simulink model "nanogrid_model"  (R2022a)
settings: Solver=VariableStepAuto  StartTime=0.0  StopTime=86000  RelTol=1e-3
undefined symbols (not defined in the file): Ion, Lithium, sigbuilder_block
libraries: spsCurrentMeasurementLib x18, spsControlledCurrentSourceLib x16, spsVoltageMeasurementLib x12, spsParallelRLCBranchLib x2, spsVariableResistorLib x2, spsBatteryLib x2, spsPVArrayLib x2, spsControlledVoltageSourceLib x1, spsSeriesRLCBranchLib x1, spspowerguiLib x1
(part 2 of 2)

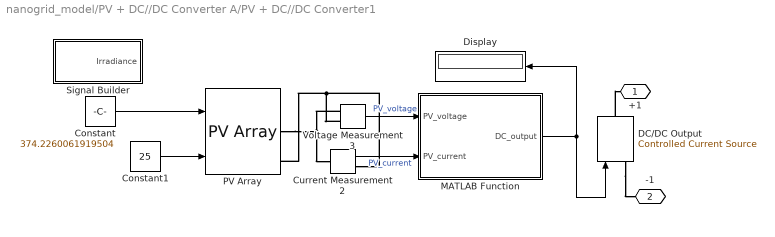
== system nanogrid_model/PV + DC//DC Converter A/PV + DC//DC Converter1 ==
  Constant : Constant  Value=374.2260061919504
  Constant1 : Constant  Value=25
  Current Measurement2 : spsCurrentMeasurementLib/Current Measurement  PhasorSimulation=off  OutputType=Complex  PSBequivalent=0
  DC/DC Output : spsControlledCurrentSourceLib/Controlled Current Source  Initialize=on  Source_Type=DC  Amplitude=0  Phase=0  Frequency=0  Measurements=None
  Display : Display
  MATLAB Function : MATLAB Function  TreatAsAtomicUnit=on
  PV Array : spsPVArrayLib/PV Array  Npar=40  Nser=10  PlotType=array @ 1000 W/m2 & specified temperatures  S_vec="[ 1000  500  100 ]"  Temp_C_vec="[ 45 25  ]"  ModuleName=User-defined  PlotWhenSelected=off  Pm=213.15  Ncell=60  Voc=36.3  Isc=7.84  Vm=29  Im=7.35  beta_Voc_pc=-0.36099  alpha_Isc_pc=0.102  beta_Voc=-0.13104  alpha_Isc=0.0079968  IL=7.8654  I0=2.9273e-10  nI=0.98119  Rsh=313.0553  Rs=0.39381  RobustModel=off  RobustCellTemperature=313.3991  BAL=on  Tc=1e-6  Tfilter=5e-5
  Signal Builder : Subsystem  Tag=STV Subsys  LoadFcn=sigbuilder_block('load');  StartFcn=sigbuilder_block('start');  StopFcn=sigbuilder_block('stop');  ClipboardFcn=sigbuilder_block('clipboard');  mask(Sigbuilder block){tuvar=[0:10]}
      mask help: Simulink:masks:SigbuilderBlock_MD
      mask init:
      | if ~strcmp(get_param(bdroot(gcbh),'SimulationStatus'),'stopped') tuvar = sigbuilder_block('maskInit'); end
      settings: CopyFcn=sigbuilder_block('copy');  DeleteFcn=sigbuilder_block('delete');  ModelCloseFcn=sigbuilder_block('modelClose');  PreSaveFcn=sigbuilder_block('preSave');  PauseFcn=sigbuilder_block('pause');  ContinueFcn=sigbuilder_block('continue');  NameChangeFcn=sigbuilder_block('namechange');  OpenFcn=sigbuilder_block('open',[509.4 101.4 550.8 400.2 ]);  CloseFcn=sigbuilder_block('close');
      mask Display: plot(0, 0, 100, 100,[2, 2, 32, 32, 2], [68, 8, 8, 68, 68],[32, 2], [38, 38], [32, 19, 2],[53, 60, 44], [32, 17, 17, 2],[16, 16, 31, 31]);txt = getActiveGroup(gcbh);text(2, 100, txt,'verticalAlignment', 'top');
  Voltage Measurement3 : spsVoltageMeasurementLib/Voltage Measurement  PhasorSimulation=off  OutputType=Complex  PSBequivalent=0
  +1 : PMIOPort  Side=Right
  -1 : PMIOPort  Port=2  Side=Right
  wires:
  MATLAB Function/1(DC_output) -> DC/DC Output/1, Display/1
  Voltage Measurement3/1 -> MATLAB Function/1(PV_voltage)  "PV_voltage"
  Current Measurement2/1 -> MATLAB Function/2(PV_current)  "PV_current"
  Constant1/1 -> PV Array/2
  Constant/1 -> PV Array/1
  connections:
  DC/DC Output/LConn1 -- -1/RConn1
  PV Array/RConn1 -- Voltage Measurement3/LConn1 -- Current Measurement2/LConn1
  Current Measurement2/RConn1 -- PV Array/RConn2 -- Voltage Measurement3/LConn2
  DC/DC Output/RConn1 -- +1/RConn1

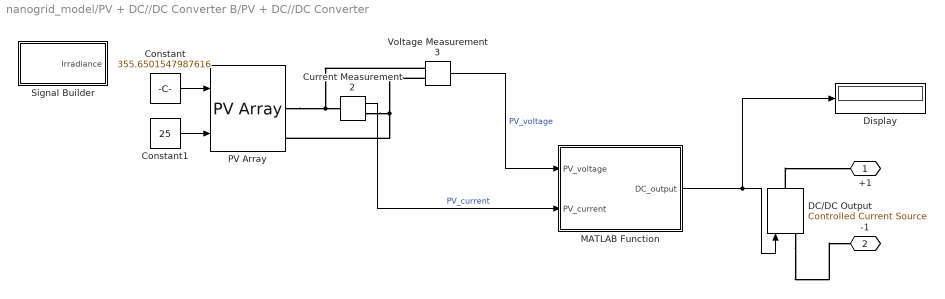
== system nanogrid_model/PV + DC//DC Converter B/PV + DC//DC Converter ==
  Constant : Constant  Value=355.6501547987616
  Constant1 : Constant  Value=25
  Current Measurement2 : spsCurrentMeasurementLib/Current Measurement  PhasorSimulation=off  OutputType=Complex  PSBequivalent=0
  DC/DC Output : spsControlledCurrentSourceLib/Controlled Current Source  Initialize=on  Source_Type=DC  Amplitude=0  Phase=0  Frequency=0  Measurements=None
  Display : Display
  MATLAB Function : MATLAB Function  TreatAsAtomicUnit=on
  PV Array : spsPVArrayLib/PV Array  Npar=40  Nser=10  PlotType=array @ 1000 W/m2 & specified temperatures  S_vec="[ 1000  500  100 ]"  Temp_C_vec="[ 45 25  ]"  ModuleName=User-defined  PlotWhenSelected=off  Pm=213.15  Ncell=60  Voc=36.3  Isc=7.84  Vm=29  Im=7.35  beta_Voc_pc=-0.36099  alpha_Isc_pc=0.102  beta_Voc=-0.13104  alpha_Isc=0.0079968  IL=7.8654  I0=2.9273e-10  nI=0.98119  Rsh=313.0553  Rs=0.39381  RobustModel=off  RobustCellTemperature=313.3991  BAL=on  Tc=1e-6  Tfilter=5e-5
  Signal Builder : Subsystem  Tag=STV Subsys  LoadFcn=sigbuilder_block('load');  StartFcn=sigbuilder_block('start');  StopFcn=sigbuilder_block('stop');  ClipboardFcn=sigbuilder_block('clipboard');  mask(Sigbuilder block){tuvar=[0:10]}
      mask help: Simulink:masks:SigbuilderBlock_MD
      mask init:
      | if ~strcmp(get_param(bdroot(gcbh),'SimulationStatus'),'stopped') tuvar = sigbuilder_block('maskInit'); end
      settings: CopyFcn=sigbuilder_block('copy');  DeleteFcn=sigbuilder_block('delete');  ModelCloseFcn=sigbuilder_block('modelClose');  PreSaveFcn=sigbuilder_block('preSave');  PauseFcn=sigbuilder_block('pause');  ContinueFcn=sigbuilder_block('continue');  NameChangeFcn=sigbuilder_block('namechange');  OpenFcn=sigbuilder_block('open',[509.4 101.4 550.8 400.2 ]);  CloseFcn=sigbuilder_block('close');
      mask Display: plot(0, 0, 100, 100,[2, 2, 32, 32, 2], [68, 8, 8, 68, 68],[32, 2], [38, 38], [32, 19, 2],[53, 60, 44], [32, 17, 17, 2],[16, 16, 31, 31]);txt = getActiveGroup(gcbh);text(2, 100, txt,'verticalAlignment', 'top');
  Voltage Measurement3 : spsVoltageMeasurementLib/Voltage Measurement  PhasorSimulation=off  OutputType=Complex  PSBequivalent=0
  +1 : PMIOPort  Side=Right
  -1 : PMIOPort  Port=2  Side=Right
  wires:
  MATLAB Function/1(DC_output) -> Display/1, DC/DC Output/1
  Voltage Measurement3/1 -> MATLAB Function/1(PV_voltage)  "PV_voltage"
  Current Measurement2/1 -> MATLAB Function/2(PV_current)  "PV_current"
  Constant1/1 -> PV Array/2
  Constant/1 -> PV Array/1
  connections:
  DC/DC Output/LConn1 -- -1/RConn1
  PV Array/RConn1 -- Voltage Measurement3/LConn1 -- Current Measurement2/LConn1
  Current Measurement2/RConn1 -- PV Array/RConn2 -- Voltage Measurement3/LConn2
  DC/DC Output/RConn1 -- +1/RConn1

== system nanogrid_model/AC+DC Load & DC//AC Converter A/AC+DC Load & DC//AC Converter1/Signal Builder ==
  Demux : Demux  Tag=STV Demux  Outputs=1
      settings: DisplayOption=none
  FromWs : FromWorkspace  Tag=STV FromWs  VariableName=tuvar
      SigBuilderData=|
      | common.afterFinalStr = 'Extrapolate'
      | common.sampleTime = 0
      | dataSet.timeRange = [0 82411]
      | dataSet.name = 'Sheet1'
      | sbobj.Groups.Name = 'Sheet1'
      | sbobj.Groups.Signals.Name = 'Load'
      | sbobj.Groups.Signals.XData = [0 3583 7166 10750 14332 17915 21498 25083 28666 32249 35832 39415 42998 46581 50164 53747 57330 60913 65000 68079 71662 75245 78828 82411]
      | sbobj.Groups.Signals.YData = [10 10 10 10 10 10 50 70 90 20 20 20 20 20 20 20 20 50 70 90 100 100 100 50]
  Load : Outport  Tag=STV Outport
  wires:
  Demux/1 -> Load/1
  FromWs/1 -> Demux/1

== system nanogrid_model/AC//DC Load & DC//AC Converter B/AC//DC Load & DC//AC Converter/Signal Builder ==
  Demux : Demux  Tag=STV Demux  Outputs=1
      settings: DisplayOption=none
  FromWs : FromWorkspace  Tag=STV FromWs  VariableName=tuvar
      SigBuilderData=|
      | common.afterFinalStr = 'Extrapolate'
      | common.sampleTime = 0
      | dataSet.timeRange = [0 82411]
      | dataSet.name = 'Sheet1'
      | sbobj.Groups.Name = 'Sheet1'
      | sbobj.Groups.Signals.Name = 'Load'
      | sbobj.Groups.Signals.XData = [0 3583 7166 10750 14332 17915 21498 25083 28666 32249 35832 39415 42998 46581 50164 53747 57330 60913 65000 68079 71662 75245 78828 82411]
      | sbobj.Groups.Signals.YData = [62 81 91 84.5 81 76 61 70 90 76.5 58 71.5 54.5 68.5 60.5 73.5 64.5 69.5 70 90 100 100 100 50]
      | sbobj.Groups.TimeRange = [0 82411]
  Load : Outport  Tag=STV Outport
  wires:
  Demux/1 -> Load/1
  FromWs/1 -> Demux/1

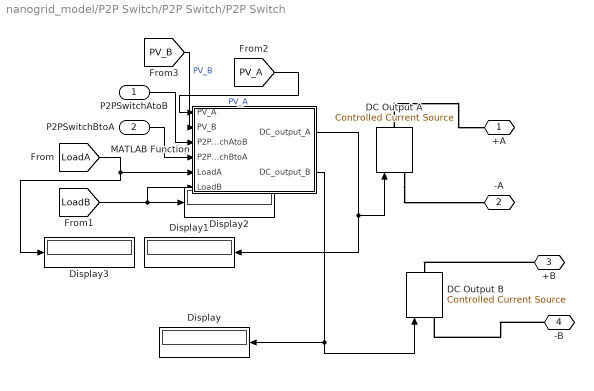
== system nanogrid_model/P2P Switch/P2P Switch/P2P Switch ==
  P2PSwitchAtoB : Inport
  P2PSwitchBtoA : Inport  Port=2
  DC Output A : spsControlledCurrentSourceLib/Controlled Current Source  Initialize=on  Source_Type=DC  Amplitude=0  Phase=0  Frequency=0  Measurements=None
  DC Output B : spsControlledCurrentSourceLib/Controlled Current Source  Initialize=on  Source_Type=DC  Amplitude=0  Phase=0  Frequency=0  Measurements=None
  Display{,1..3} (4 alike) : Display
  MATLAB Function : MATLAB Function  TreatAsAtomicUnit=on
  +A : PMIOPort  Side=Right
  -A : PMIOPort  Port=2  Side=Right
  +B : PMIOPort  Port=3  Side=Right
  -B : PMIOPort  Port=4  Side=Right
  wires:
  MATLAB Function/1(DC_output_A) -> DC Output A/1, Display1/1
  P2PSwitchAtoB/1 -> MATLAB Function/3(P2PSwitchAtoB)
  MATLAB Function/2(DC_output_B) -> Display/1, DC Output B/1
  P2PSwitchBtoA/1 -> MATLAB Function/4(P2PSwitchBtoA)
  [LoadA] -> Display3/1, MATLAB Function/5(LoadA)
  [LoadB] -> Display2/1, MATLAB Function/6(LoadB)
  [PV_A] -> MATLAB Function/1(PV_A)  "PV_A"
  [PV_B] -> MATLAB Function/2(PV_B)  "PV_B"
  connections:
  DC Output A/LConn1 -- -A/RConn1
  DC Output A/RConn1 -- +A/RConn1
  +B/RConn1 -- DC Output B/RConn1
  -B/RConn1 -- DC Output B/LConn1

== system nanogrid_model/PV + DC//DC Converter A/PV + DC//DC Converter1/Signal Builder ==
  Demux : Demux  Tag=STV Demux  Outputs=1
      settings: DisplayOption=none
  FromWs : FromWorkspace  Tag=STV FromWs  VariableName=tuvar
      SigBuilderData=|
      | common.afterFinalStr = 'Extrapolate'
      | common.sampleTime = 0
      | dataSet.timeRange = [0 82411]
      | dataSet.name = 'Sheet1'
      | sbobj.Groups.Name = 'Sheet1'
      | sbobj.Groups.Signals.Name = 'Irradiance'
      | sbobj.Groups.Signals.XData = [0 3583 7166 10750 14332 17915 21498 25083 28666 32249 35832 39415 42998 46581 50164 53747 57330 60913 65000 68079 71662 75245 78828 82411]
      | sbobj.Groups.Signals.YData = [0 0 0 0 0 0 0 100 200 300 400 500 600 500 400 300 200 100 0 0 0 0 0 0]
      | sbobj.Groups.TimeRange = [0 86000]
  Irradiance : Outport  Tag=STV Outport
  wires:
  Demux/1 -> Irradiance/1
  FromWs/1 -> Demux/1

== system nanogrid_model/PV + DC//DC Converter B/PV + DC//DC Converter/Signal Builder ==
  Demux : Demux  Tag=STV Demux  Outputs=1
      settings: DisplayOption=none
  FromWs : FromWorkspace  Tag=STV FromWs  VariableName=tuvar
      SigBuilderData=|
      | common.afterFinalStr = 'Extrapolate'
      | common.sampleTime = 0
      | dataSet.timeRange = [0 82411]
      | dataSet.name = 'Sheet1'
      | sbobj.Groups.Name = 'Sheet1'
      | sbobj.Groups.Signals.Name = 'Irradiance'
      | sbobj.Groups.Signals.XData = [0 3583 7166 10750 14332 17915 21498 25083 28666 32249 35832 39415 42998 46581 50164 53747 57330 60913 65000 68079 71662 75245 78828 82411]
      | sbobj.Groups.Signals.YData = [0 0 0 0 0 0 0 100 200 300 400 500 600 500 400 300 200 100 0 0 0 0 0 0]
      | sbobj.Groups.TimeRange = [0 86000]
  Irradiance : Outport  Tag=STV Outport
  wires:
  Demux/1 -> Irradiance/1
  FromWs/1 -> Demux/1

== stateflow chart nanogrid_model/Stateflow Algorithm A ==
  state PurchaseEnergy
    exit:
    switchUtilityPurchase=0;
    P2PPurchaseRequest=0;
    state Utilitygrid
      entry:
      currentState = "PUG";
    state NanoGrid
      entry:
      currentState = "PNG";
    PurchaseEnergy.Utilitygrid -> (junction 309) : [DERPrice<=gridPrice || gridOutage]
    (junction 309) -> PurchaseEnergy.Utilitygrid [order 2] : {P2PPurchaseRequest=0;switchUtilityPurchase=1;}
    (junction 310) -> PurchaseEnergy.Utilitygrid [order 1] : [~P2PEnergyTrading]{switchUtilityPurchase=1;}
    (default) -> (junction 307)
    (junction 307) -> (junction 309)
    (junction 310) -> (junction 309) [order 3]
    (junction 308) -> (junction 310) : {P2PPurchaseRequest=1;}
    (junction 309) -> (junction 308) [order 1] : [DERPrice <= gridPrice || gridOutage]
    PurchaseEnergy.NanoGrid -> (junction 309) : [~P2PEnergyTrading||DERPrice>gridPrice]
    (junction 310) -> PurchaseEnergy.NanoGrid [order 2] : [P2PEnergyTrading]{switchUtilityPurchase=0;}
  state SellEnergy
    exit:
    switchUtilitySell=0;
    P2PSaleRequest=0;
    state Utilitygrid
      entry:
      currentState = "SUG";
    state NanoGrid
      entry:
      currentState = "SNG";
    (junction 325) -> SellEnergy.Utilitygrid [order 2] : {P2PSaleRequest=0;switchUtilitySell=1;}
    SellEnergy.Utilitygrid -> (junction 325) : [gridOutage||DERPrice>=feedInTariff]
    (junction 324) -> SellEnergy.Utilitygrid [order 2] : [~P2PEnergyTrading]{switchUtilitySell=1;}
    (default) -> (junction 317)
    (junction 317) -> (junction 325)
    (junction 324) -> (junction 325) [order 3]
    (junction 325) -> (junction 316) [order 1] : [DERPrice >= feedInTariff || gridOutage]
    (junction 316) -> (junction 324) : {P2PSaleRequest=1;}
    SellEnergy.NanoGrid -> (junction 325) : [~P2PEnergyTrading||DERPrice<feedInTariff]
    (junction 324) -> SellEnergy.NanoGrid [order 1] : [P2PEnergyTrading]{switchUtilitySell=0;}
  state SelfConsumption
    state GeneratorMode
      entry:
      currentState = "GM"
      switchGenerator = 1;
      exit:
      switchGenerator = 0;
    state RenewableSources
      entry:
      currentState = "PV"
    (default) -> (junction 281)
    (junction 281) -> GeneratorMode [order 1] : [SOC<=1]
    (junction 281) -> RenewableSources [order 2]
  (default) -> (junction 290)
  (junction 290) -> PurchaseEnergy [order 1] : [SOC<20 && SOC>1]
  (junction 290) -> SellEnergy [order 2] : [SOC>80]
  PurchaseEnergy -> (junction 290) : [SOC>=20 || SOC < 1]
  SellEnergy -> (junction 290) : [SOC<=80]
  SelfConsumption -> (junction 290) : [SOC>80 || SOC<80 && SOC > 1]
  (junction 290) -> SelfConsumption [order 3]
  data: gridOutage input; SOC input; currentState output; DERPrice input; feedInTariff input; switchGenerator output; gridPrice input; switchUtilityPurchase output; switchUtilitySell output; P2PEnergyTrading input; P2PPurchaseRequest output; P2PSaleRequest output

== matlab function nanogrid_model/AC//DC Converter B/MATLAB Function ==
  data: switchGridPurchase input; switchGridSell input; gridOutage input; DC_output output; AC_output output; LoadB input; PV_B input
function [DC_output,AC_output] = fcn(switchGridPurchase, switchGridSell, gridOutage, LoadB, PV_B)

dischargeCurrent = 217;
chargeCurrent = 217;
lowChargeCRate = 0.1;
converterEfficiencyLoss = 0.95;

if(gridOutage)
    DC_output = 0;
    AC_output = 0;
elseif(switchGridSell)
    DC_output = -(dischargeCurrent+PV_B)*converterEfficiencyLoss;
    AC_output = (dischargeCurrent+PV_B)*sqrt(2)*converterEfficiencyLoss;
elseif(switchGridPurchase)
    DC_output = (chargeCurrent*lowChargeCRate+(-LoadB)-PV_B)*converterEfficiencyLoss*1.1;
    AC_output = (-chargeCurrent*lowChargeCRate+(-LoadB)-PV_B)*converterEfficiencyLoss*1.1;
else
    DC_output = 0;
    AC_output = 0; 
end
end

== stateflow chart nanogrid_model/Stateflow Algorithm B ==
  state PurchaseEnergy
    exit:
    switchUtilityPurchase=0;
    P2PPurchaseRequest=0;
    state Utilitygrid
      entry:
      currentState = "PUG";
    state NanoGrid
      entry:
      currentState = "PNG";
    PurchaseEnergy.Utilitygrid -> (junction 705) : [DERPrice<=gridPrice || gridOutage]
    (junction 705) -> PurchaseEnergy.Utilitygrid [order 2] : {P2PPurchaseRequest=0;switchUtilityPurchase=1;}
    (junction 702) -> PurchaseEnergy.Utilitygrid [order 1] : [~P2PEnergyTrading]{switchUtilityPurchase=1;}
    (default) -> (junction 704)
    (junction 704) -> (junction 705)
    (junction 702) -> (junction 705) [order 3]
    (junction 700) -> (junction 702) : {P2PPurchaseRequest=1;}
    (junction 705) -> (junction 700) [order 1] : [DERPrice <= gridPrice || gridOutage]
    PurchaseEnergy.NanoGrid -> (junction 705) : [~P2PEnergyTrading||DERPrice>gridPrice]
    (junction 702) -> PurchaseEnergy.NanoGrid [order 2] : [P2PEnergyTrading]{switchUtilityPurchase=0;}
  state SellEnergy
    exit:
    switchUtilitySell=0;
    P2PSaleRequest=0;
    state Utilitygrid
      entry:
      currentState = "SUG";
    state NanoGrid
      entry:
      currentState = "SNG";
    (junction 726) -> SellEnergy.Utilitygrid [order 2] : {P2PSaleRequest=0;switchUtilitySell=1;}
    SellEnergy.Utilitygrid -> (junction 726) : [gridOutage||DERPrice>=feedInTariff]
    (junction 742) -> SellEnergy.Utilitygrid [order 2] : [~P2PEnergyTrading]{switchUtilitySell=1;}
    (default) -> (junction 740)
    (junction 740) -> (junction 726)
    (junction 742) -> (junction 726) [order 3]
    (junction 726) -> (junction 738) [order 1] : [DERPrice >= feedInTariff || gridOutage]
    (junction 738) -> (junction 742) : {P2PSaleRequest=1;}
    SellEnergy.NanoGrid -> (junction 726) : [~P2PEnergyTrading||DERPrice<feedInTariff]
    (junction 742) -> SellEnergy.NanoGrid [order 1] : [P2PEnergyTrading]{switchUtilitySell=0;}
  state SelfConsumption
    state GeneratorMode
      entry:
      currentState = "GM"
      switchGenerator = 1;
      exit:
      switchGenerator = 0;
    state RenewableSources
      entry:
      currentState = "PV"
    (default) -> (junction 724)
    (junction 724) -> GeneratorMode [order 1] : [SOC<=1]
    (junction 724) -> RenewableSources [order 2]
  (default) -> (junction 744)
  (junction 744) -> PurchaseEnergy [order 1] : [SOC<20 && SOC>1]
  (junction 744) -> SellEnergy [order 2] : [SOC>80]
  PurchaseEnergy -> (junction 744) : [SOC>=20 || SOC < 1]
  SellEnergy -> (junction 744) : [SOC<=80]
  SelfConsumption -> (junction 744) : [SOC>80 || SOC<80 && SOC > 1]
  (junction 744) -> SelfConsumption [order 3]
  data: gridOutage input; SOC input; currentState output; DERPrice input; feedInTariff input; switchGenerator output; gridPrice input; P2PPurchaseRequest output; P2PSaleRequest output; switchUtilityPurchase output; switchUtilitySell output; P2PEnergyTrading input

== matlab function nanogrid_model/PV + DC//DC Converter B/PV + DC//DC Converter/MATLAB Function ==
  data: PV_voltage input; PV_current input; DC_output output
function DC_output = fcn(PV_voltage, PV_current)

converterEfficiencyLoss = 0.95;

DC_output = PV_current*converterEfficiencyLoss;


end

== matlab function nanogrid_model/Backup Gas Generator + DC//DC Converter B/Backup Gas Generator + DC//DC Converter/MATLAB Function ==
  data: switchGenerator input; Gen_voltage input; Gen_current input; DC_output output; DC_output_Gen output
function [DC_output,DC_output_Gen] = fcn(switchGenerator, Gen_voltage, Gen_current)

converterEfficiencyLoss = 0.95;

if(switchGenerator)
    DC_output_Gen = 200*converterEfficiencyLoss;
else
    DC_output_Gen = 0;
end
DC_output = DC_output_Gen*converterEfficiencyLoss;

== matlab function nanogrid_model/AC//DC Load & DC//AC Converter B/AC//DC Load & DC//AC Converter/MATLAB Function ==
  data: DC_voltage input; DC_current input; AC_output output
function AC_output = fcn(DC_voltage, DC_current)

converterEfficiencyLoss = 0.95;
DC_power = DC_current * DC_voltage;

AC_output = sqrt(2)*converterEfficiencyLoss*DC_current; 

end

== matlab function nanogrid_model/P2P Switch/P2P Switch/P2P Switch/MATLAB Function ==
  data: PV_A input; PV_B input; P2PSwitchAtoB input; DC_output_A output; DC_output_B output; P2PSwitchBtoA input; LoadA input; LoadB input
function [DC_output_A, DC_output_B] = fcn(PV_A, PV_B, P2PSwitchAtoB,P2PSwitchBtoA, LoadA, LoadB)

chargeCurrent = 217;
lowChargeCRate = 0.1;%low c-rates extend battery life cycles
converterEfficiencyLoss = 0.95;

if(P2PSwitchAtoB)
    DC_output_A = -(chargeCurrent*lowChargeCRate*1.1+(-LoadB)-PV_B)*converterEfficiencyLoss;%subtraction of nano grid member b's PV is due to the battery's charge limitation (whatever is produced by the PV does not need to be drawn from A's battery, if the total power would exceed the maximum battery charge current)
    DC_output_B = (chargeCurrent*lowChargeCRate*1.1+(-LoadB)-PV_B)*converterEfficiencyLoss;
elseif(P2PSwitchBtoA)
    DC_output_A = (chargeCurrent*lowChargeCRate*1.1+(-LoadA)-PV_A)*converterEfficiencyLoss;%current must be at least sufficient to supply the load otherwise the battery won't charge
    DC_output_B = -(chargeCurrent*lowChargeCRate*1.1+(-LoadA)-PV_A)*converterEfficiencyLoss;
else
    DC_output_A = 0;
    DC_output_B = 0;
end

== matlab function nanogrid_model/AC//DC Converter A/MATLAB Function ==
  data: switchGridPurchase input; switchGridSell input; DC_output output; AC_output output; gridOutage input; LoadA input; PV_A input
function [DC_output,AC_output] = fcn(switchGridPurchase, switchGridSell, gridOutage, LoadA, PV_A)

dischargeCurrent = 217;
chargeCurrent = 217;
lowChargeCRate = 0.1;
converterEfficiencyLoss = 0.95;

if(gridOutage)
    DC_output = 0;
    AC_output = 0;
elseif(switchGridSell)
    DC_output = -(dischargeCurrent+PV_A);
    AC_output = (dischargeCurrent+PV_A)*sqrt(2);
elseif(switchGridPurchase)
    DC_output = (chargeCurrent*lowChargeCRate*1.1+(-LoadA)-PV_A)*converterEfficiencyLoss;
    AC_output = (-chargeCurrent*lowChargeCRate*1.1+(-LoadA)-PV_A)*converterEfficiencyLoss;
else
    DC_output = 0;
    AC_output = 0; 
end
end

== matlab function nanogrid_model/Backup Gas Generator + DC//DC Converter A/Backup Gas Generator + DC//DC Converter1/MATLAB Function ==
  data: switchGenerator input; DC_output output; DC_output_Gen output
function [DC_output,DC_output_Gen] = fcn(switchGenerator)

converterEfficiencyLoss = 0.95;

if(switchGenerator)
    DC_output_Gen = 200*converterEfficiencyLoss;
else
    DC_output_Gen = 0;
end
DC_output = DC_output_Gen*converterEfficiencyLoss;

== matlab function nanogrid_model/PV + DC//DC Converter A/PV + DC//DC Converter1/MATLAB Function ==
  data: PV_voltage input; PV_current input; DC_output output
function DC_output = fcn(PV_voltage, PV_current)

converterEfficiencyLoss = 0.95;

DC_output = PV_current*converterEfficiencyLoss;


end

== matlab function nanogrid_model/AC+DC Load & DC//AC Converter A/AC+DC Load & DC//AC Converter1/MATLAB Function ==
  data: DC_voltage input; DC_current input; AC_output output
function AC_output = fcn(DC_voltage, DC_current)

converterEfficiencyLoss = 0.95;
DC_power = DC_current * DC_voltage;

AC_output = sqrt(2)*converterEfficiencyLoss*DC_current; 

end
